simulink model "power_aircraft_distribution_mexido_V2"  (R2014b)
settings: Solver=ode45  StartTime=0.0  StopTime=.1  RelTol=1e-3
libraries: powerlib x8, sps_avr x1, powerlib_meascontrol x1
settings Model: Creator=JPSOLIV  LastModifiedBy=JPSOLIV

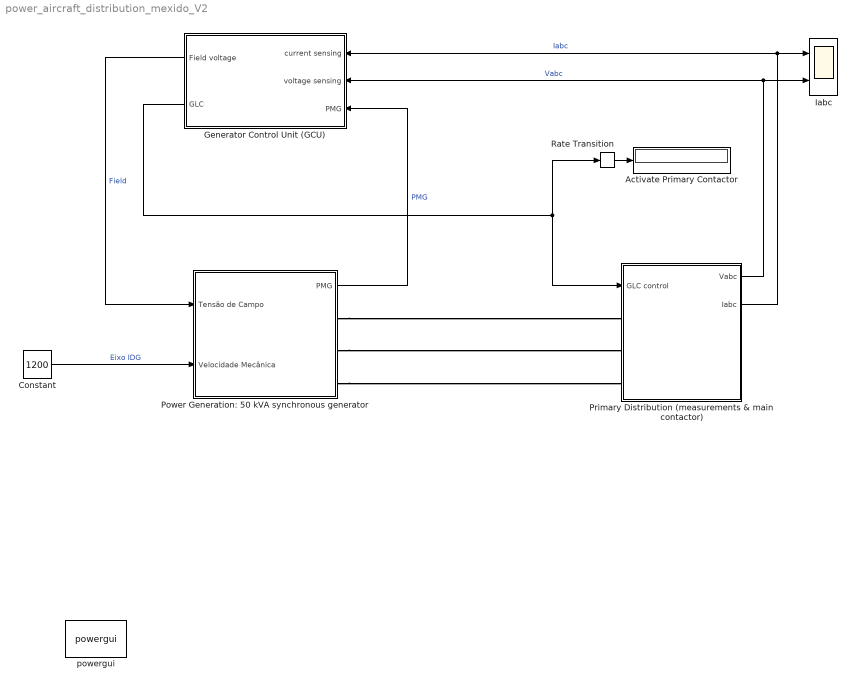
== system power_aircraft_distribution_mexido_V2 ==
  Activate Primary Contactor : Display
      settings: SampleTime=1e-2
  Constant : Constant  Value=1200
  Generator Control Unit (GCU) : Subsystem
      mask Display: image(imread('power_aircraft_distribution_GCU.jpg','jpg'))
  Iabc : Scope  NumInputPorts=2
      settings: YMin=-1~-5e+156  YMax=1~5e+156
  Power Generation: 50 kVA synchronous generator : Subsystem
      mask Display: image(imread('power_aircraft_distribution_APU_Generator.jpg','jpg'))
  Primary Distribution (measurements & main contactor) : Subsystem
  Rate Transition : RateTransition  OutPortSampleTimeOpt=Inherit  OutPortSampleTime=Ts
  powergui : powerlib/powergui  Priority=1  SimulationMode=Discrete  SolverType=Tustin/Backward Euler (TBE)  SampleTime=5e-7  frequency=60  SPID=off  DisableSnubberDevices=off  DisableRonSwitches=off  DisableVfSwitches=off  SwTol=0  DisplayEquations=off  Interpol=off  methode=off  Ts=100  frequencyindice=0  Pbase=100e6  ErrMax=1e-4  Iterations=50  UnitsV=kV  UnitsW=MW  FunctionMessages=off  echomessages=off  HookPort=off  EnableUseOfTLC=off  x0status=blocks  RestoreLinks=warning  ResistiveCurrentMeasurement=off  Frange=[0:2:500]  Ylog=off  Xlog=on  ShowGrid=off  save=off  variable=ZData  structure=0  ZoomFFT=off  StartTime=0.0  cycles=1  DisplayStyle=1  fundamental=60  FreqAxis=off  MaxFrequency=1000  frequencyindicesteady=1  RmsSteady=1  display=off
  wires:
  Power Generation: 50 kVA synchronous generator/1(PMG) -> Generator Control Unit (GCU)/3(PMG)  "PMG"
  Generator Control Unit (GCU)/1(Field voltage) -> Power Generation: 50 kVA synchronous generator/1(Tensão de Campo)  "Field"
  Primary Distribution (measurements & main contactor)/1(Vabc) -> Iabc/2, Generator Control Unit (GCU)/2(voltage sensing)  "Vabc"
  Primary Distribution (measurements & main contactor)/2(Iabc) -> Iabc/1, Generator Control Unit (GCU)/1(current sensing)  "Iabc"
  Generator Control Unit (GCU)/2(GLC) -> Rate Transition/1, Primary Distribution (measurements & main contactor)/1(GLC control)
  Constant/1 -> Power Generation: 50 kVA synchronous generator/2("Velocidade Mecânica ")  "Eixo IDG"
  Rate Transition/1 -> Activate Primary Contactor/1
  connections:
  Power Generation: 50 kVA synchronous generator/RConn3 -- Primary Distribution (measurements & main contactor)/LConn3
  Power Generation: 50 kVA synchronous generator/RConn2 -- Primary Distribution (measurements & main contactor)/LConn2
  Power Generation: 50 kVA synchronous generator/RConn1 -- Primary Distribution (measurements & main contactor)/LConn1

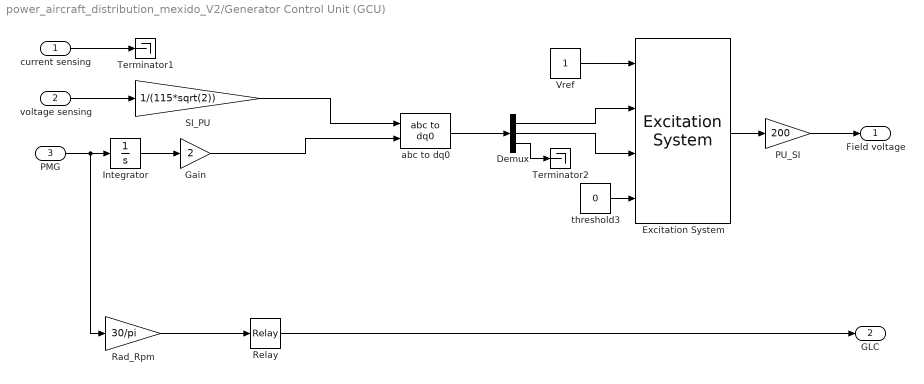
== system power_aircraft_distribution_mexido_V2/Generator Control Unit (GCU) ==
  current sensing : Inport
  voltage sensing : Inport  Port=2
  PMG : Inport  Port=3
  Demux : Demux  Outputs=3
  Excitation System : sps_avr/Excitation System  tr=20e-3  reg=[ 300, 0.001 ]  exc=[ 1, 0 ]  tgr=[ 0, 0 ]  damp=[ 0.001, 0.1 ]  sat=[ 0, 0 ]  lim=[ -2, 2, 0 ]  v0=[1 0]
  Gain : Gain  Gain=2
  Integrator : Integrator
  PU_SI : Gain  Gain=200
  Rad_Rpm : Gain  Gain=30/pi
  Relay : Relay  OnSwitchValue=9000  OffSwitchValue=8900
  SI_PU : Gain  Gain=1/(115*sqrt(2))
  Terminator1 : Terminator
  Terminator2 : Terminator
  Vref : Constant
  abc to dq0 : powerlib_meascontrol/Transformations/abc to dq0  Alignment=90 degrees behind phase A axis
  threshold3 : Constant  Value=0
  Field voltage : Outport
  GLC : Outport  Port=2
  wires:
  Relay/1 -> GLC/1
  Demux/3 -> Terminator2/1
  current sensing/1 -> Terminator1/1
  threshold3/1 -> Excitation System/4
  Vref/1 -> Excitation System/1
  Rad_Rpm/1 -> Relay/1
  PU_SI/1 -> Field voltage/1
  Excitation System/1 -> PU_SI/1
  SI_PU/1 -> abc to dq0/1
  Demux/2 -> Excitation System/3
  Demux/1 -> Excitation System/2
  abc to dq0/1 -> Demux/1
  Integrator/1 -> Gain/1
  voltage sensing/1 -> SI_PU/1
  PMG/1 -> Rad_Rpm/1, Integrator/1
  Gain/1 -> abc to dq0/2

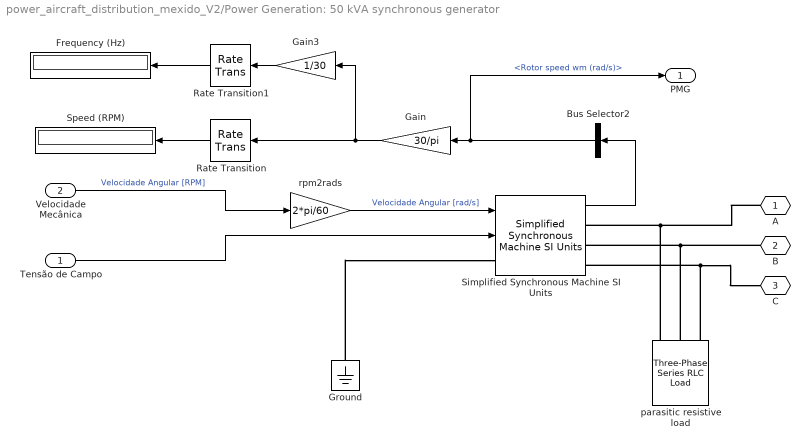
== system power_aircraft_distribution_mexido_V2/Power Generation: 50 kVA synchronous generator ==
  Tensão de Campo : Inport
  "Velocidade Mecânica " : Inport  Port=2
  Bus Selector2 : BusSelector  OutputSignals=Rotor speed wm (rad/s)
  Frequency (Hz) : Display
      settings: SampleTime=1e-2
  Gain : Gain  Gain=30/pi
  Gain3 : Gain  Gain=1/30
  Ground : powerlib/Elements/Ground  LConnTagsString=a
  Rate Transition : RateTransition  OutPortSampleTimeOpt=Inherit  OutPortSampleTime=Ts
  Rate Transition1 : RateTransition  OutPortSampleTimeOpt=Inherit  OutPortSampleTime=Ts
  Simplified Synchronous Machine SI Units : powerlib/Machines/Simplified Synchronous Machine SI Units  ConnectionType=4-wire Y  MechanicalLoad=Speed w  MeasurementBus=off  NominalParameters=[50e3 115*sqrt(3) 400]  Mechanical=[0.02 0 4]  InternalRL="[0.0204  0.08104e-3]"  InitialConditions=[-99,0 0,0,0 0,0,0]  Units=1  LoadFlowParameters=[1,0,0,0,0]  TsPowergui=0  TsBlock=Ts  BusType=PV  Pref=0  Qref=0  Qmin=-inf  Qmax=+inf  PLF=0  QLF=0
  Speed (RPM) : Display
      settings: SampleTime=1e-2
  parasitic resistive load : powerlib/Elements/Three-Phase Series RLC Load  LConnTagsString=A|B|C  Configuration=Y (grounded)  NominalVoltage=115  NominalFrequency=400  ActivePower=5000  InductivePower=0  CapacitivePower=0  Measurements=None  LoadType=constant Z
  rpm2rads : Gain  Gain=2*pi/60
  A : PMIOPort  Tag=PMCPort  Port=1  Side=Right
  B : PMIOPort  Tag=PMCPort  Port=2  Side=Right
  C : PMIOPort  Tag=PMCPort  Port=3  Side=Right
  PMG : Outport
  wires:
  Simplified Synchronous Machine SI Units/1 -> Bus Selector2/1
  Tensão de Campo/1 -> Simplified Synchronous Machine SI Units/2
  Bus Selector2/1 -> Gain/1, PMG/1  "<Rotor speed wm (rad/s)>"
  Gain/1 -> Gain3/1, Rate Transition/1
  Gain3/1 -> Rate Transition1/1
  "Velocidade Mecânica "/1 -> rpm2rads/1  "Velocidade Angular [RPM]"
  rpm2rads/1 -> Simplified Synchronous Machine SI Units/1  "Velocidade Angular [rad/s]"
  Rate Transition/1 -> Speed (RPM)/1
  Rate Transition1/1 -> Frequency (Hz)/1
  connections:
  A/RConn1 -- parasitic resistive load/LConn1 -- Simplified Synchronous Machine SI Units/RConn1
  B/RConn1 -- parasitic resistive load/LConn2 -- Simplified Synchronous Machine SI Units/RConn2
  parasitic resistive load/LConn3 -- C/RConn1 -- Simplified Synchronous Machine SI Units/RConn3
  Ground/LConn1 -- Simplified Synchronous Machine SI Units/LConn1

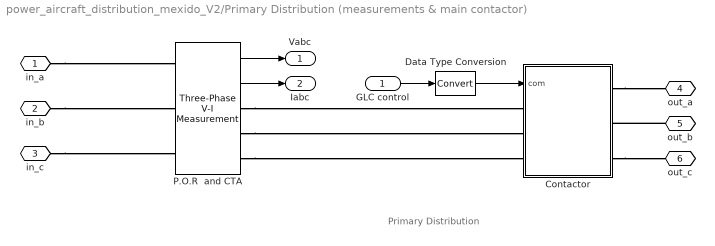
== system power_aircraft_distribution_mexido_V2/Primary Distribution (measurements & main contactor) ==
  note: Primary Distribution
  GLC control : Inport
  Contactor : Subsystem
  Data Type Conversion : DataTypeConversion
  P.O.R  and CTA : powerlib/Measurements/Three-Phase V-I Measurement  VoltageMeasurement=phase-to-ground  SetLabelV=off  LabelV=Vabc  Vpu=off  VpuLL=off  CurrentMeasurement=yes  SetLabelI=off  LabelI=Iabc  Ipu=off  Pbase=100e6  Vbase=500e3  OutputType=Complex  PhasorSimulation=off  PSBequivalent=0
  in_a : PMIOPort  Port=1  Side=Left
  in_b : PMIOPort  Port=2  Side=Left
  in_c : PMIOPort  Port=3  Side=Left
  out_a : PMIOPort  Port=4  Side=Right
  out_b : PMIOPort  Port=5  Side=Right
  out_c : PMIOPort  Port=6  Side=Right
  Vabc : Outport
  Iabc : Outport  Port=2
  wires:
  GLC control/1 -> Data Type Conversion/1
  P.O.R  and CTA/1 -> Vabc/1
  P.O.R  and CTA/2 -> Iabc/1
  Data Type Conversion/1 -> Contactor/1(com)
  connections:
  in_a/RConn1 -- P.O.R  and CTA/LConn1
  in_b/RConn1 -- P.O.R  and CTA/LConn2
  in_c/RConn1 -- P.O.R  and CTA/LConn3
  P.O.R  and CTA/RConn1 -- Contactor/LConn1
  P.O.R  and CTA/RConn2 -- Contactor/LConn2
  P.O.R  and CTA/RConn3 -- Contactor/LConn3
  Contactor/RConn1 -- out_a/RConn1
  out_b/RConn1 -- Contactor/RConn2
  Contactor/RConn3 -- out_c/RConn1

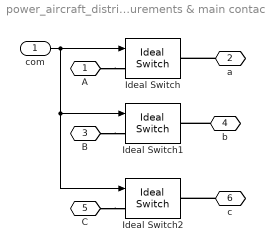
== system power_aircraft_distribution_mexido_V2/Primary Distribution (measurements & main contactor)/Contactor ==
  com : Inport
  Ideal Switch : powerlib/Power Electronics/Ideal Switch  Ron=0.001  Lon=0  IC=0  Rs=1e3  Cs=inf  Measurements=off
  Ideal Switch1 : powerlib/Power Electronics/Ideal Switch  Ron=0.001  Lon=0  IC=0  Rs=1e3  Cs=inf  Measurements=off
  Ideal Switch2 : powerlib/Power Electronics/Ideal Switch  Ron=0.001  Lon=0  IC=0  Rs=1e3  Cs=inf  Measurements=off
  A : PMIOPort  Port=1  Side=Left
  a : PMIOPort  Port=2  Side=Right
  B : PMIOPort  Port=3  Side=Left
  b : PMIOPort  Port=4  Side=Right
  C : PMIOPort  Port=5  Side=Left
  c : PMIOPort  Port=6  Side=Right
  wires:
  com/1 -> Ideal Switch1/1, Ideal Switch2/1, Ideal Switch/1
  connections:
  c/RConn1 -- Ideal Switch2/RConn1
  C/RConn1 -- Ideal Switch2/LConn1
  b/RConn1 -- Ideal Switch1/RConn1
  B/RConn1 -- Ideal Switch1/LConn1
  a/RConn1 -- Ideal Switch/RConn1
  A/RConn1 -- Ideal Switch/LConn1
